simulink model "RTP_V37"  (R2020b)
settings: Solver=VariableStepAuto  StartTime=0.0  StopTime=40  RelTol=1e-3
settings Model: Creator=barac  LastModifiedBy=barac

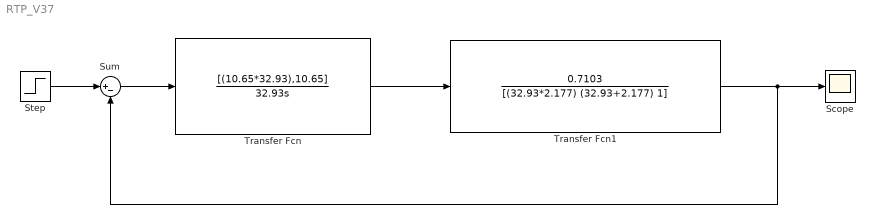
== system RTP_V37 ==
  Scope : Scope
  Step : Step  SampleTime=0
  Sum : Sum  Inputs=|+-
  Transfer Fcn : TransferFcn  Numerator=[(10.65*32.93),10.65]  Denominator=[32.93 0]
  Transfer Fcn1 : TransferFcn  Numerator=[0.7103]  Denominator=[(32.93*2.177) (32.93+2.177) 1]
  wires:
  Transfer Fcn/1 -> Transfer Fcn1/1
  Step/1 -> Sum/1
  Sum/1 -> Transfer Fcn/1
  Transfer Fcn1/1 -> Sum/2, Scope/1
